simulink model "Test_Harness"  (R2018b)
settings: Solver=FixedStepAuto  StartTime=0  StopTime=300  MaxStep=0.01  RelTol=1e-4  EnableMultiTasking=on
undefined symbols (not defined in the file): actuatorCentres, aeroCoeff, datcom1, deflectionLimits, HDBK, MIL, sensorSampleTime, vehicle
libraries: arduinolib x7, aerolibasang x5, aerolibactuator x4, aerolibadyn x3, aerolibconvert2 x2, shared6dof x1, aerolibwind2 x1, aerolibatmos2 x1, pil_lib x1, aerolibanimutils x1
settings Model: DataDictionary=data.sldd  VariantConfigurationObject=Variants  SnapshotBufferSize=2  SnapshotInterval=1  PacingRate=10  ExtModeTrigDuration=2  Creator=Aliak  LastModifiedBy=Aliak
settings SolverCC: SolverResetMethod=Robust  MinimalZcImpactIntegration=on
settings OptimizationCC: DefaultParameterBehavior=Inlined  UseDivisionForNetSlopeComputation=on  UseFloatMulNetSlope=on  DefaultUnderspecifiedDataType=single  UseSpecifiedMinMax=on  InlineInvariantSignals=on  EnhancedBackFolding=on  BooleansAsBitfields=on  PassReuseOutputArgsAs=Individual arguments  StateBitsets=on  DataBitsets=on  ZeroExternalMemoryAtStartup=off  ZeroInternalMemoryAtStartup=off  NoFixptDivByZeroProtection=on  EfficientFloat2IntCast=on  LifeSpan=0.01  MaxStackSize=64  SimCompilerOptimization=on  OptimizeBlockOrder=speed  DifferentSizesBufferReuse=on
settings DebuggingCC: ConsistencyChecking=warning  ReadBeforeWriteMsg=DisableAll  WriteAfterWriteMsg=DisableAll  WriteAfterReadMsg=DisableAll  SolverPrmCheckMsg=warning  ParameterTunabilityLossMsg=error  UniqueDataStoreMsg=error  BusObjectLabelMismatch=error  StateNameClashWarn=warning  ForceCombineOutputUpdateInSim=on
settings HardwareCC: ProdBitPerInt=16  ProdBitPerPointer=16  ProdBitPerSizeT=16  ProdBitPerPtrDiffT=16  ProdLargestAtomicFloat=None  ProdWordSize=8  ProdLongLongMode=on  ProdHWDeviceType=Atmel->AVR
settings ModelReferenceCC: UpdateModelReferenceTargets=IfOutOfDate  EnableParallelModelReferenceBuilds=on  ModelReferenceMinAlgLoopOccurrences=on
settings SFSimCC: SimUserIncludeDirs="\"nativelibs/include\" \"nativelibs/src\" \"nativelibs/build\""  SFSimEcho=off  MATLABDynamicMemAlloc=off
settings RTWCC: SystemTargetFile=ert.tlc  HardwareBoard=Arduino Uno  TemplateMakefile=ert_default_tmf  GenerateReport=on  RTWUseSimCustomCode=on  CustomInclude="\"nativelibs/include\" \"nativelibs/src\" \"nativelibs/build\""  Toolchain=Arduino AVR  BuildConfiguration=Faster Runs  IncludeHyperlinkInReport=on  LaunchReport=on  PortableWordSizes=on  CreateSILPILBlock=PIL  GenerateTraceInfo=on  GenerateTraceReport=on  GenerateTraceReportSl=on  GenerateTraceReportSf=on  GenerateTraceReportEml=on  GenerateCodeMetricsReport=on
settings CodeAppCC: ForceParamTrailComments=on  IgnoreCustomStorageClasses=off  OperatorAnnotations=on  SimulinkDataObjDesc=on  SFDataObjDesc=on  CustomSymbolStrGlobalVar=rt$N$M  CustomSymbolStrType=$N$M  CustomSymbolStrFcn=$N$M$F  CustomSymbolStrMacro=$N$M  InsertBlockDesc=on
settings ERTTargetCC: TargetLangStandard=C99 (ISO)  UtilityFuncGeneration=Shared location  IncludeMdlTerminateFcn=off  CombineSignalStateStructs=on  SuppressErrorStatus=on  SupportNonFinite=off  SupportComplex=off  SupportVariableSizeSignals=on  CastingMode=Standards  ERTFilePackagingFormat=CompactWithDataFile

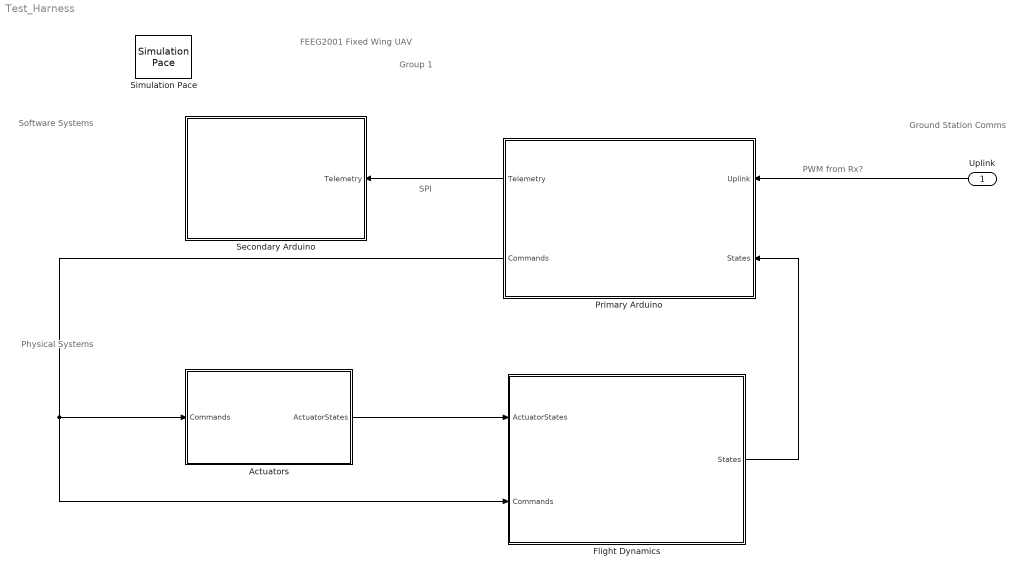
== system Test_Harness ==
  note: PWM from Rx?
  note: SPI
  note: Group 1
  note: FEEG2001 Fixed Wing UAV
  note: Physical Systems
  note: Software Systems
  note: Ground Station Comms
  Uplink : Inport  OutDataTypeStr=Bus: Uplink
  Actuators : Subsystem  Variant=on
  Flight Dynamics : Subsystem
      mask Display: image('MQ-9-Reaper-armed-UAV.jpg');
  Primary Arduino : Subsystem  DialogController=pil_create_dialog  LoadFcn=|
      | try
      |    if ~strcmp(rtw.pil.getPILVersion, '9.5 (R2018b)_13')
      |       set_param(gcb, 'DialogController', '');
      |       set_param(gcb, 'DialogControllerArgs', '');
      |    end
      | catch e
      |       set_param(gcb, 'DialogController', '');
      |       set_param(gcb, 'DialogControllerArgs', '');
      | end
      mask help: PIL:pil:XILBlockMaskDesc
      mask Display: disp('PIL');
  Secondary Arduino : Subsystem  VariantControl=Variant1
      mask Display: image('a000066_featured_1_.jpg');
  Simulation Pace : aerolibanimutils/Simulation Pace  SimulationPace=1  SleepMode=Auto  OutputPaceError=off  SampleTime=sensorSampleTime
  wires:
  Actuators/1(ActuatorStates) -> Flight Dynamics/1(ActuatorStates)
  Primary Arduino/2(Commands) -> Flight Dynamics/2(Commands), Actuators/1(Commands)
  Uplink/1 -> Primary Arduino/1(Uplink)
  Flight Dynamics/1(States) -> Primary Arduino/2(States)
  Primary Arduino/1(Telemetry) -> Secondary Arduino/1(Telemetry)

== system Test_Harness/Actuators ==
  Commands : Inport
  Model Actuators : Subsystem  VariantControl=SimType == 0
  Real Actuators : Subsystem  VariantControl=SimType == 1
  ActuatorStates : Outport

== system Test_Harness/Flight Dynamics ==
  ActuatorStates : Inport
  Commands : Inport  Port=2  OutDataTypeStr=Bus: Commands
  6DOF EOM : Subsystem  VariantControl=eom3DOF
  Bus Selector : BusSelector  OutputSignals=Throttle
  Coeff Model : Subsystem  Commented=on  VariantControl=AeroModel==2
  DATCOM Model : Subsystem  VariantControl=AeroModel==1
  Environment : Subsystem
  Propulsion : Subsystem
      settings: RTWSystemCode=Inline
  Sum1 : Sum  Inputs=|++  SaturateOnIntegerOverflow=on  InputSameDT=on  OutDataTypeStr=Inherit: Same as first input
  Sum2 : Sum  Inputs=|++  SaturateOnIntegerOverflow=on  InputSameDT=on  OutDataTypeStr=Inherit: Same as first input
  Visualization : Subsystem
  States : Outport
  wires:
  Commands/1 -> Bus Selector/1
  Sum2/1 -> 6DOF EOM/2(Forces)
  Propulsion/1(F) -> Sum2/2
  Propulsion/2(M) -> Sum1/2
  Sum1/1 -> 6DOF EOM/3(Moments)
  Bus Selector/1 -> Propulsion/1(cmd)  "<Throttle>"
  ActuatorStates/1 -> DATCOM Model/3(ActuatorStates)
  DATCOM Model/1(F) -> Sum2/1
  DATCOM Model/2(M) -> Sum1/1
  Environment/1(Env) -> 6DOF EOM/1(Env), DATCOM Model/1(Env)
  6DOF EOM/1(DCMbe) -> Environment/2(DCMbe)
  6DOF EOM/2(States) -> Environment/1(States), Visualization/1(States), DATCOM Model/2(States), States/1

== system Test_Harness/Primary Arduino ==
  Uplink : Inport  OutDataTypeStr=Bus: Uplink
  States : Inport  Port=2
  Primary Arduino_sfcn : pil_lib/PIL Block  SimulationMode=PIL  IsTopModelPIL=off  CodeDir=D:\MATLABProjects\FEEG2001-FWUAV\libs\Primary_ert_rtw  AnchorDir=D:\MATLABProjects\FEEG2001-FWUAV\libs  ConfigName=Arduino Board  XrelIsTopModelCode=on  XrelIsReusable=off  XrelDWorkNames={}  XrelDWorkTypes={}  XrelModelArgVals={}  XrelOrderedParamNames={}
  __InputSSForSFun__ : Subsystem
  __OutputSSForSFun__ : Subsystem
  Telemetry : Outport  OutDataTypeStr=Bus: Sensors  SampleTime=[1 0]
  Commands : Outport  Port=2  OutDataTypeStr=Bus: Commands  SampleTime=[-1 0]
  wires:
  Uplink/1 -> __InputSSForSFun__/1(Uplink)
  States/1 -> __InputSSForSFun__/2(States)
  __InputSSForSFun__/1(__UniqueOutportName__1__) -> Primary Arduino_sfcn/1
  __InputSSForSFun__/2(__UniqueOutportName__2__) -> Primary Arduino_sfcn/2
  __InputSSForSFun__/3(__UniqueOutportName__3__) -> Primary Arduino_sfcn/3
  __InputSSForSFun__/4(__UniqueOutportName__4__) -> Primary Arduino_sfcn/4
  __InputSSForSFun__/5(__UniqueOutportName__5__) -> Primary Arduino_sfcn/5
  __InputSSForSFun__/6(__UniqueOutportName__6__) -> Primary Arduino_sfcn/6
  __InputSSForSFun__/7(__UniqueOutportName__7__) -> Primary Arduino_sfcn/7
  Primary Arduino_sfcn/1 -> __OutputSSForSFun__/1(__UniqueInportName__1__)
  Primary Arduino_sfcn/2 -> __OutputSSForSFun__/2(__UniqueInportName__2__)
  __OutputSSForSFun__/1(Telemetry) -> Telemetry/1
  __OutputSSForSFun__/2(Commands) -> Commands/1

== system Test_Harness/Secondary Arduino ==
  Telemetry : Inport
  Telemetry Logging : Subsystem  VariantControlMode=Label  Variant=on  VariantControl=Variant1  LabelModeActiveChoice=SecArd==0
  wires:
  Telemetry/1 -> Telemetry Logging/1("Telemetry ")

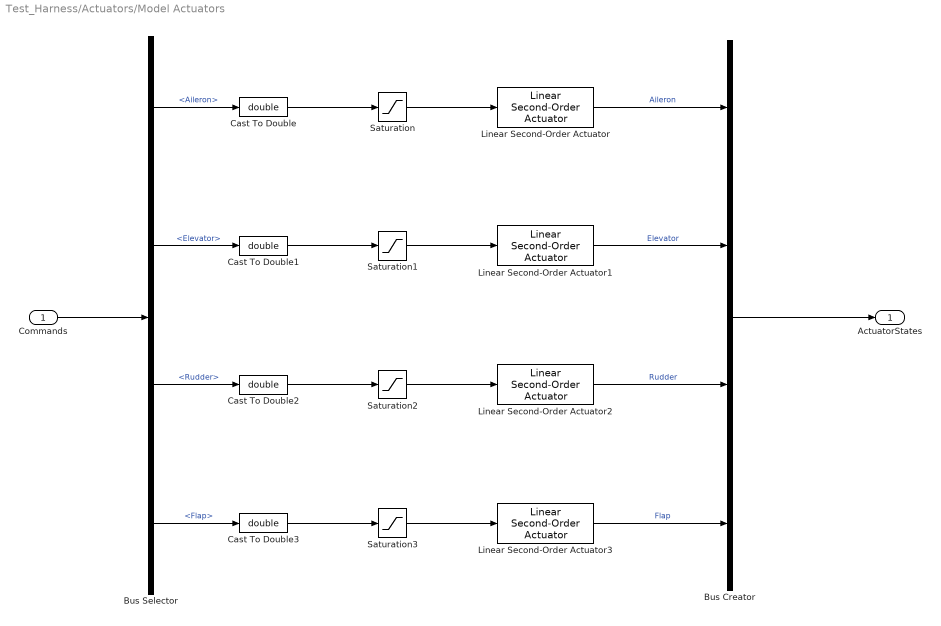
== system Test_Harness/Actuators/Model Actuators ==
  Commands : Inport
  Bus Creator : BusCreator  Inputs=4  OutDataTypeStr=Bus: ActuatorStates
  Bus Selector : BusSelector  OutputSignals=Aileron,Elevator,Rudder,Flap
  Cast To Double{,1..3} (4 alike) : DataTypeConversion  OutDataTypeStr=double
  Linear Second-Order Actuator{,1..3} (4 alike) : aerolibactuator/Linear Second-Order Actuator  wn_fin=1  z_fin=0.3  fin_act_0=0  fin_act_vel=0
      settings: SourceProductName=Aerospace Blockset  SourceProductBaseCode=AE
  Saturation : Saturate  UpperLimit=deflectionLimits.aileron.max  LowerLimit=deflectionLimits.aileron.min
  Saturation1 : Saturate  UpperLimit=deflectionLimits.elevator.max  LowerLimit=deflectionLimits.elevator.min
  Saturation2 : Saturate  UpperLimit=deflectionLimits.rudder.max  LowerLimit=deflectionLimits.rudder.min
  Saturation3 : Saturate  UpperLimit=deflectionLimits.flap.max  LowerLimit=deflectionLimits.flap.min
  ActuatorStates : Outport
  wires:
  Bus Selector/3 -> Cast To Double2/1  "<Rudder>"
  Bus Selector/4 -> Cast To Double3/1  "<Flap>"
  Bus Selector/1 -> Cast To Double/1  "<Aileron>"
  Bus Selector/2 -> Cast To Double1/1  "<Elevator>"
  Saturation/1 -> Linear Second-Order Actuator/1
  Saturation1/1 -> Linear Second-Order Actuator1/1
  Saturation2/1 -> Linear Second-Order Actuator2/1
  Saturation3/1 -> Linear Second-Order Actuator3/1
  Linear Second-Order Actuator1/1 -> Bus Creator/2  "Elevator"
  Linear Second-Order Actuator/1 -> Bus Creator/1  "Aileron"
  Linear Second-Order Actuator2/1 -> Bus Creator/3  "Rudder"
  Linear Second-Order Actuator3/1 -> Bus Creator/4  "Flap"
  Bus Creator/1 -> ActuatorStates/1
  Commands/1 -> Bus Selector/1
  Cast To Double/1 -> Saturation/1
  Cast To Double1/1 -> Saturation1/1
  Cast To Double2/1 -> Saturation2/1
  Cast To Double3/1 -> Saturation3/1

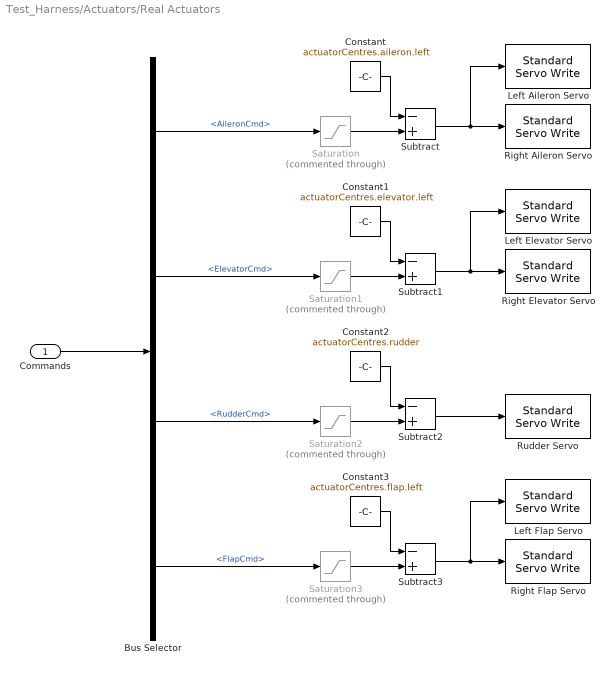
== system Test_Harness/Actuators/Real Actuators ==
  Commands : Inport
  Bus Selector : BusSelector  OutputSignals=AileronCmd,ElevatorCmd,RudderCmd,FlapCmd
  Constant : Constant  Value=actuatorCentres.aileron.left
  Constant1 : Constant  Value=actuatorCentres.elevator.left
  Constant2 : Constant  Value=actuatorCentres.rudder
  Constant3 : Constant  Value=actuatorCentres.flap.left
  Left Aileron Servo : arduinolib/Standard Servo Write  pinNumber=servoPins.aileron.left  ServoIndex=0  blockPlatform=ARDUINO
      settings: SourceProductName=Simulink Support Package for Arduino Hardware
  Left Elevator Servo : arduinolib/Standard Servo Write  pinNumber=servoPins.elevator.left  ServoIndex=0  blockPlatform=ARDUINO
      settings: SourceProductName=Simulink Support Package for Arduino Hardware
  Left Flap Servo : arduinolib/Standard Servo Write  pinNumber=servoPins.flap.left  ServoIndex=0  blockPlatform=ARDUINO
      settings: SourceProductName=Simulink Support Package for Arduino Hardware
  Right Aileron Servo : arduinolib/Standard Servo Write  pinNumber=servoPins.aileron.right  ServoIndex=0  blockPlatform=ARDUINO
      settings: SourceProductName=Simulink Support Package for Arduino Hardware
  Right Elevator Servo : arduinolib/Standard Servo Write  pinNumber=servoPins.elevator.right  ServoIndex=0  blockPlatform=ARDUINO
      settings: SourceProductName=Simulink Support Package for Arduino Hardware
  Right Flap Servo : arduinolib/Standard Servo Write  pinNumber=servoPins.flap.right  ServoIndex=0  blockPlatform=ARDUINO
      settings: SourceProductName=Simulink Support Package for Arduino Hardware
  Rudder Servo : arduinolib/Standard Servo Write  pinNumber=servoPins.rudder  ServoIndex=0  blockPlatform=ARDUINO
      settings: SourceProductName=Simulink Support Package for Arduino Hardware
  Saturation : Saturate  Commented=through  UpperLimit=deflectionLimits.aileron.max  LowerLimit=deflectionLimits.aileron.min
  Saturation1 : Saturate  Commented=through  UpperLimit=deflectionLimits.elevator.max  LowerLimit=deflectionLimits.elevator.min
  Saturation2 : Saturate  Commented=through  UpperLimit=deflectionLimits.rudder.max  LowerLimit=deflectionLimits.rudder.min
  Saturation3 : Saturate  Commented=through  UpperLimit=deflectionLimits.flap.max  LowerLimit=deflectionLimits.flap.min
  Subtract{,1..3} (4 alike) : Sum  Inputs=-+
  wires:
  Saturation/1 -> Subtract/2
  Bus Selector/3 -> Saturation2/1  "<RudderCmd>"
  Commands/1 -> Bus Selector/1
  Bus Selector/4 -> Saturation3/1  "<FlapCmd>"
  Subtract3/1 -> Right Flap Servo/1, Left Flap Servo/1
  Bus Selector/1 -> Saturation/1  "<AileronCmd>"
  Constant2/1 -> Subtract2/1
  Subtract2/1 -> Rudder Servo/1
  Saturation3/1 -> Subtract3/2
  Saturation2/1 -> Subtract2/2
  Saturation1/1 -> Subtract1/2
  Bus Selector/2 -> Saturation1/1  "<ElevatorCmd>"
  Subtract/1 -> Right Aileron Servo/1, Left Aileron Servo/1
  Subtract1/1 -> Right Elevator Servo/1, Left Elevator Servo/1
  Constant/1 -> Subtract/1
  Constant1/1 -> Subtract1/1
  Constant3/1 -> Subtract3/1

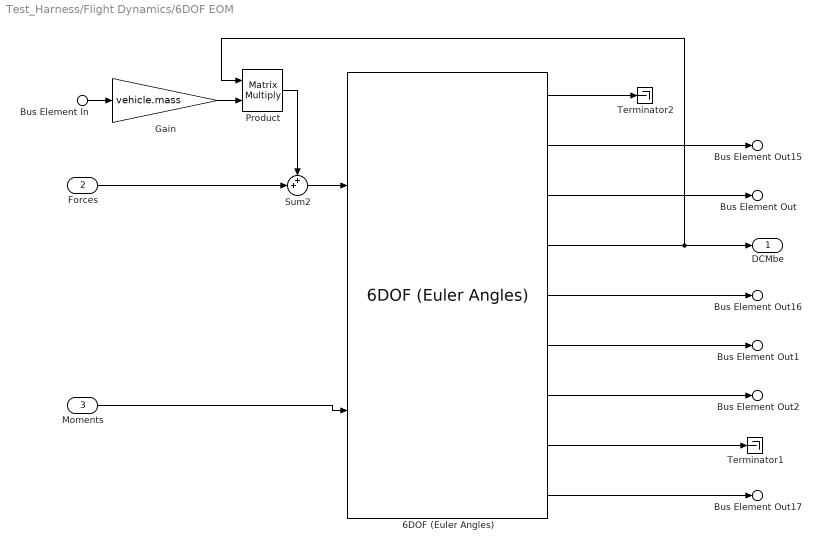
== system Test_Harness/Flight Dynamics/6DOF EOM ==
  Bus Element In : Inport  PortName=Env  Element=g
  Forces : Inport  Port=2
  Moments : Inport  Port=3
  6DOF (Euler Angles) : shared6dof/6DOF (Euler Angles)  units=Metric (MKS)  mtype=Fixed  rep=Euler Angles  xme_0=initConditions.x0  Vm_0=initConditions.v0  eul_0=initConditions.euler0  pm_0=initConditions.w0  mass_0=vehicle.mass  mass_e=0.5  mass_f=2.0  inertia=vehicle.inertia  inertia_e=eye(3)  inertia_f=2*eye(3)  k_quat=1.0  vre_flag=on  abi_flag=on  aMode=0  xme_statename=''  Vm_statename=''  eul_statename=''  quat_statename=''  pm_statename=''  mass_statename=''
      settings: SourceProductBaseCode=AE
  Gain : Gain  Gain=vehicle.mass
  Product : Product  Multiplication=Matrix(*)
  Sum2 : Sum  Inputs=++|  SaturateOnIntegerOverflow=on  InputSameDT=on  OutDataTypeStr=Inherit: Same as first input
  Terminator1 : Terminator
  Terminator2 : Terminator
  DCMbe : Outport
  Bus Element Out : Outport  Port=2  PortName=States  Element=phi_theta_psi
  Bus Element Out1 : Outport  Port=2  PortName=States  Element=pqr
  Bus Element Out2 : Outport  Port=2  PortName=States  Element=omega_dot
  Bus Element Out15 : Outport  Port=2  PortName=States  Element=X_e
  Bus Element Out16 : Outport  Port=2  PortName=States  Element=V_b
  Bus Element Out17 : Outport  Port=2  PortName=States  Element=A_be
  wires:
  6DOF (Euler Angles)/4 -> DCMbe/1, Product/1
  6DOF (Euler Angles)/1 -> Terminator2/1
  Bus Element In/1 -> Gain/1
  6DOF (Euler Angles)/9 -> Bus Element Out17/1
  6DOF (Euler Angles)/7 -> Bus Element Out2/1
  6DOF (Euler Angles)/6 -> Bus Element Out1/1
  6DOF (Euler Angles)/5 -> Bus Element Out16/1
  6DOF (Euler Angles)/3 -> Bus Element Out/1
  6DOF (Euler Angles)/2 -> Bus Element Out15/1
  Gain/1 -> Product/2
  Sum2/1 -> 6DOF (Euler Angles)/1
  Product/1 -> Sum2/1
  6DOF (Euler Angles)/8 -> Terminator1/1
  Moments/1 -> 6DOF (Euler Angles)/2
  Forces/1 -> Sum2/2

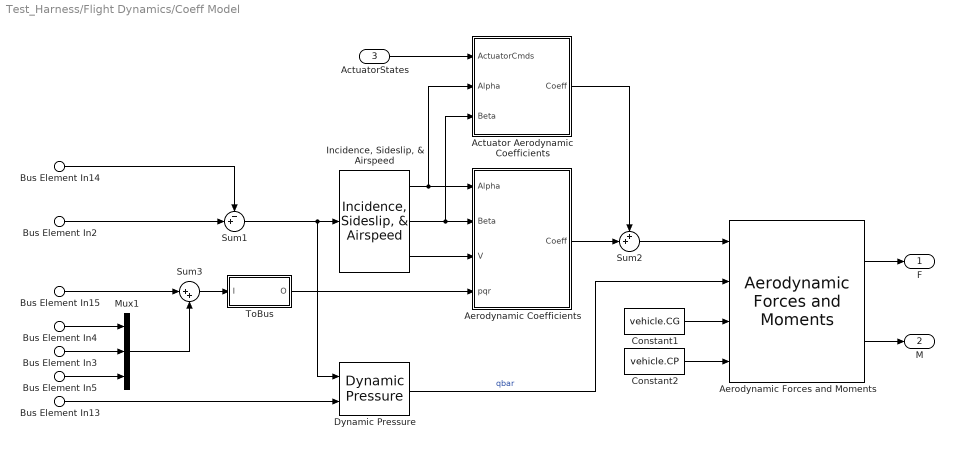
== system Test_Harness/Flight Dynamics/Coeff Model ==
  Bus Element In13 : Inport  PortName=Env  Element=AirDensity
  Bus Element In14 : Inport  PortName=Env  Element=WindVelocity
  Bus Element In15 : Inport  PortName=Env  Element=WindAngularRates
  Bus Element In3 : Inport  Port=2  PortName=States  Element=q
  Bus Element In4 : Inport  Port=2  PortName=States  Element=p
  Bus Element In5 : Inport  Port=2  PortName=States  Element=r
  Bus Element In2 : Inport  Port=2  PortName=States  Element=V_b
  ActuatorStates : Inport  Port=3  OutDataTypeStr=Bus: ActuatorStates
  Actuator Aerodynamic Coefficients : Subsystem
  Aerodynamic Coefficients : Subsystem
  Aerodynamic Forces and Moments : aerolibadyn/Aerodynamic Forces and Moments   inputAxes=Body  outputForceAxes=Body  outputMomentAxes=Body  S=vehicle.wingarea  b=vehicle.wingspan  cbar=vehicle.aclength
      settings: SourceProductName=Aerospace Blockset
  Constant1 : Constant  Value=vehicle.CG
  Constant2 : Constant  Value=vehicle.CP
  Dynamic Pressure : aerolibasang/Dynamic Pressure
  "Incidence, Sideslip, & Airspeed" : aerolibasang/Incidence, Sideslip, & Airspeed
      settings: SourceProductName=Aerospace Blockset
  Mux1 : Mux  Inputs=3
  Sum1 : Sum  Inputs=-+|  SaturateOnIntegerOverflow=on  InputSameDT=on  OutDataTypeStr=Inherit: Same as first input
  Sum2 : Sum  Inputs=++|
  Sum3 : Sum  Inputs=|++  SaturateOnIntegerOverflow=on  InputSameDT=on  OutDataTypeStr=Inherit: Same as first input
  ToBus : Subsystem
  F : Outport  Unit=N
  M : Outport  Port=2  Unit=N*m
  wires:
  ActuatorStates/1 -> Actuator Aerodynamic Coefficients/1(ActuatorCmds)
  Bus Element In14/1 -> Sum1/1
  Bus Element In2/1 -> Sum1/2
  Mux1/1 -> Sum3/2
  Bus Element In15/1 -> Sum3/1
  Bus Element In5/1 -> Mux1/3
  Bus Element In3/1 -> Mux1/2
  Bus Element In4/1 -> Mux1/1
  Actuator Aerodynamic Coefficients/1(Coeff) -> Sum2/1
  Aerodynamic Coefficients/1(Coeff) -> Sum2/2
  ToBus/1(O) -> Aerodynamic Coefficients/4(pqr)
  Sum1/1 -> Dynamic Pressure/1, "Incidence, Sideslip, & Airspeed"/1
  Dynamic Pressure/1 -> Aerodynamic Forces and Moments/2  "qbar"
  Sum3/1 -> ToBus/1(I)
  Bus Element In13/1 -> Dynamic Pressure/2
  "Incidence, Sideslip, & Airspeed"/3 -> Aerodynamic Coefficients/3(V)
  "Incidence, Sideslip, & Airspeed"/2 -> Aerodynamic Coefficients/2(Beta), Actuator Aerodynamic Coefficients/3(Beta)
  Aerodynamic Forces and Moments/2 -> M/1
  Aerodynamic Forces and Moments/1 -> F/1
  Constant2/1 -> Aerodynamic Forces and Moments/4
  Constant1/1 -> Aerodynamic Forces and Moments/3
  Sum2/1 -> Aerodynamic Forces and Moments/1
  "Incidence, Sideslip, & Airspeed"/1 -> Actuator Aerodynamic Coefficients/2(Alpha), Aerodynamic Coefficients/1(Alpha)

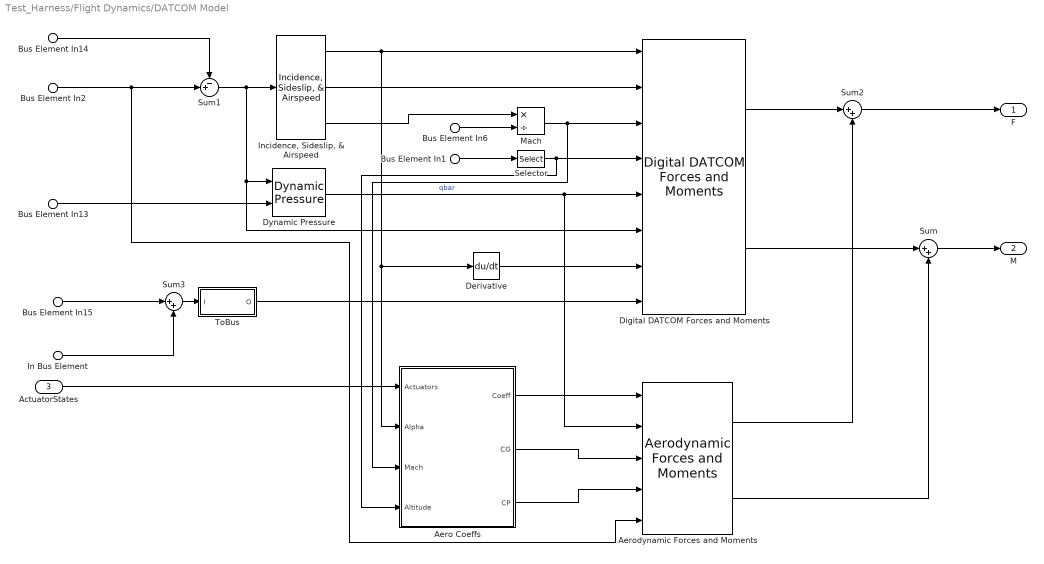
== system Test_Harness/Flight Dynamics/DATCOM Model ==
  Bus Element In13 : Inport  PortName=Env  Element=AirDensity
  Bus Element In14 : Inport  PortName=Env  Element=WindVelocity
  Bus Element In15 : Inport  PortName=Env  Element=WindAngularRates
  Bus Element In6 : Inport  PortName=Env  Element=a
  Bus Element In2 : Inport  Port=2  PortName=States  Element=V_b
  Bus Element In1 : Inport  Port=2  PortName=States  Element=X_e
  In Bus Element : Inport  Port=2  PortName=States  Element=pqr
  ActuatorStates : Inport  Port=3  OutDataTypeStr=Bus: ActuatorStates
  Aero Coeffs : Subsystem
  "Aerodynamic Forces and Moments " : aerolibadyn/Aerodynamic Forces and Moments   inputAxes=Stability  outputForceAxes=Body  outputMomentAxes=Body  S=vehicle.wingarea  b=vehicle.wingspan  cbar=vehicle.cbar
      settings: SourceProductName=Aerospace Blockset
  Derivative : Derivative
  Digital DATCOM Forces and Moments : aerolibadyn/Digital DATCOM Forces and Moments  units=Metric (MKS)  dcase=datcom1{3}  fmode=Body  buildno=0  imethod=Linear  emethod=Linear  rmethod=Linear Extrapolation  action=Warning
      settings: SourceProductName=Aerospace Blockset  SourceProductBaseCode=AE
  Dynamic Pressure : aerolibasang/Dynamic Pressure
  "Incidence, Sideslip, & Airspeed" : aerolibasang/Incidence, Sideslip, & Airspeed
      settings: SourceProductName=Aerospace Blockset
  Mach : Product  Inputs=*/
  Selector : Selector  IndexMode=Zero-based  InputPortWidth=3  IndexOptions=Index vector (dialog)  Indices=[2]  OutputSizes=1
  Sum : Sum  Inputs=|++
  Sum1 : Sum  Inputs=-+|  SaturateOnIntegerOverflow=on  InputSameDT=on  OutDataTypeStr=Inherit: Same as first input
  Sum2 : Sum  Inputs=|++
  Sum3 : Sum  Inputs=|++  SaturateOnIntegerOverflow=on  InputSameDT=on  OutDataTypeStr=Inherit: Same as first input
  ToBus : Subsystem
  F : Outport  Unit=N
  M : Outport  Port=2  Unit=N*m
  wires:
  Bus Element In14/1 -> Sum1/1
  Bus Element In2/1 -> "Aerodynamic Forces and Moments "/5, Sum1/2
  In Bus Element/1 -> Sum3/2
  Bus Element In15/1 -> Sum3/1
  Sum1/1 -> "Incidence, Sideslip, & Airspeed"/1, Digital DATCOM Forces and Moments/6, Dynamic Pressure/1
  Sum3/1 -> ToBus/1(I)
  Bus Element In13/1 -> Dynamic Pressure/2
  "Incidence, Sideslip, & Airspeed"/3 -> Mach/1
  Digital DATCOM Forces and Moments/2 -> Sum/1
  Digital DATCOM Forces and Moments/1 -> Sum2/1
  Dynamic Pressure/1 -> "Aerodynamic Forces and Moments "/2, Digital DATCOM Forces and Moments/5  "qbar"
  Bus Element In1/1 -> Selector/1
  Selector/1 -> Aero Coeffs/4(Altitude), Digital DATCOM Forces and Moments/4
  Bus Element In6/1 -> Mach/2
  ActuatorStates/1 -> Aero Coeffs/1(Actuators)
  "Incidence, Sideslip, & Airspeed"/2 -> Digital DATCOM Forces and Moments/2
  "Incidence, Sideslip, & Airspeed"/1 -> Digital DATCOM Forces and Moments/1, Derivative/1, Aero Coeffs/2(Alpha)
  Aero Coeffs/1(Coeff) -> "Aerodynamic Forces and Moments "/1
  Aero Coeffs/2(CG) -> "Aerodynamic Forces and Moments "/3
  Aero Coeffs/3(CP) -> "Aerodynamic Forces and Moments "/4
  Sum/1 -> M/1
  "Aerodynamic Forces and Moments "/2 -> Sum/2
  Sum2/1 -> F/1
  "Aerodynamic Forces and Moments "/1 -> Sum2/2
  ToBus/1(O) -> Digital DATCOM Forces and Moments/8
  Derivative/1 -> Digital DATCOM Forces and Moments/7
  Mach/1 -> Digital DATCOM Forces and Moments/3, Aero Coeffs/3(Mach)

== system Test_Harness/Flight Dynamics/Environment ==
  States : Inport
  DCMbe : Inport  Port=2
  Bus Creator : BusCreator  Inputs=5
  Bus Selector : BusSelector  OutputSignals=X_e,V_b
  Dryden Wind Turbulence Model (Discrete (-q +r)) : aerolibwind2/Dryden Wind Turbulence Model  (Continuous (+q -r))  units=Metric (MKS)  spec=MIL-HDBK-1797  model=Discrete Dryden (-q +r)  W20=1  Wdeg=250  TurbProb=10^-1  L_high=533.4  Wingspan=1.8  ts=sensorSampleTime  Seed=[23341 23342 23343 23344]  T_on=off
      settings: SourceProductName=Aerospace Blockset
  Lapse Rate Model : aerolibatmos2/ISA Atmosphere Model  custom=off  g=9.80665  gamma=1.4  R=287.0531  L=0.0065  h_trop=11000  h_strat=20000  rho0=1.225  P0=101325  T0=288.15  h0=0
      settings: SourceProductName=Aerospace Blockset
  Selector : Selector  IndexMode=Zero-based  InputPortWidth=3  IndexOptions=Index vector (dialog)  Indices=[0]  OutputSizes=1
  Selector1 : Selector  IndexMode=Zero-based  InputPortWidth=3  IndexOptions=Index vector (dialog)  Indices=[0]  OutputSizes=1
  Terminator : Terminator
  Terminator1 : Terminator
  g : Constant  Value=[0 0 9.80665]
  Env : Outport
  wires:
  States/1 -> Bus Selector/1
  Bus Creator/1 -> Env/1
  Selector/1 -> Dryden Wind Turbulence Model (Discrete (-q +r))/1, Lapse Rate Model/1
  Bus Selector/1 -> Selector/1  "<X_e>"
  Lapse Rate Model/4 -> Bus Creator/2  "AirDensity"
  Lapse Rate Model/2 -> Bus Creator/1  "a"
  g/1 -> Bus Creator/3  "g"
  DCMbe/1 -> Dryden Wind Turbulence Model (Discrete (-q +r))/3
  Bus Selector/2 -> Selector1/1  "<V_b>"
  Selector1/1 -> Dryden Wind Turbulence Model (Discrete (-q +r))/2
  Dryden Wind Turbulence Model (Discrete (-q +r))/1 -> Bus Creator/4  "WindVelocity"
  Dryden Wind Turbulence Model (Discrete (-q +r))/2 -> Bus Creator/5  "WindAngularRates"
  Lapse Rate Model/1 -> Terminator/1
  Lapse Rate Model/3 -> Terminator1/1

== system Test_Harness/Flight Dynamics/Propulsion ==
  cmd : Inport  OutDataTypeStr=single
  Cast To Double : DataTypeConversion  OutDataTypeStr=double
  Mux : Mux  Inputs=[1 2]
  Product : Product
  ThrustX : Lookup_n-D  NumberOfTableDimensions=1  LookupTableObject=''  BreakpointsForDimension1=(1/6)*(3+([-3:3]))  IndexSearchMethod=Linear search  BeginIndexSearchUsingPreviousIndexResult=on  Table=vehicle.thrust*(1+tanh([-3:3]))  ExtrapMethod=Clip  InternalRulePriority=Speed
  ThrustYZ : Constant  Value=[0 0]'  SampleTime=-1
  Thrust_M1 : Constant  Value=[-0.1 0 0.01]  SampleTime=-1
  Vector Concatenate : Concatenate
  F : Outport  Unit=N
  M : Outport  Port=2  Unit=N*m
  wires:
  Thrust_M1/1 -> Product/2
  ThrustX/1 -> Mux/1, Vector Concatenate/2
  ThrustYZ/1 -> Vector Concatenate/1, Mux/2
  Mux/1 -> F/1
  cmd/1 -> Cast To Double/1
  Product/1 -> M/1
  Vector Concatenate/1 -> Product/1
  Cast To Double/1 -> ThrustX/1

== system Test_Harness/Flight Dynamics/Visualization ==
  Bus Element In3 : Inport  PortName=States  Element=pqr
  Bus Element In9 : Inport  PortName=States  Element=X_e
  In Bus Element : Inport  PortName=States  Element=V_b
  In Bus Element1 : Inport  PortName=States  Element=phi_theta_psi
  "Incidence, Sideslip, & Airspeed" : aerolibasang/Incidence, Sideslip, & Airspeed
      settings: SourceProductName=Aerospace Blockset
  Mux5 : Mux  Inputs=2
  State Plots : Scope  NumInputPorts=4
  Terminator : Terminator
  wires:
  Bus Element In9/1 -> State Plots/4
  In Bus Element1/1 -> State Plots/2
  Mux5/1 -> State Plots/1
  "Incidence, Sideslip, & Airspeed"/2 -> Mux5/2  "beta"
  "Incidence, Sideslip, & Airspeed"/1 -> Mux5/1  "alpha"
  In Bus Element/1 -> "Incidence, Sideslip, & Airspeed"/1
  Bus Element In3/1 -> State Plots/3
  "Incidence, Sideslip, & Airspeed"/3 -> Terminator/1

== system Test_Harness/Primary Arduino/__InputSSForSFun__ ==
  Uplink : Inport  OutDataTypeStr=Bus: Uplink
  States : Inport  Port=2
  temporaryBusSelectName_1 : BusSelector  OutputSignals=phi_theta_psi,pqr,omega_dot,X_e,V_b,A_be
  __UniqueOutportName__1__ : Outport
  __UniqueOutportName__2__ : Outport  Port=2
  __UniqueOutportName__3__ : Outport  Port=3
  __UniqueOutportName__4__ : Outport  Port=4
  __UniqueOutportName__5__ : Outport  Port=5
  __UniqueOutportName__6__ : Outport  Port=6
  __UniqueOutportName__7__ : Outport  Port=7
  wires:
  States/1 -> temporaryBusSelectName_1/1
  Uplink/1 -> __UniqueOutportName__1__/1
  temporaryBusSelectName_1/1 -> __UniqueOutportName__2__/1  "<phi_theta_psi>"
  temporaryBusSelectName_1/2 -> __UniqueOutportName__3__/1  "<pqr>"
  temporaryBusSelectName_1/3 -> __UniqueOutportName__4__/1  "<omega_dot>"
  temporaryBusSelectName_1/4 -> __UniqueOutportName__5__/1  "<X_e>"
  temporaryBusSelectName_1/5 -> __UniqueOutportName__6__/1  "<V_b>"
  temporaryBusSelectName_1/6 -> __UniqueOutportName__7__/1  "<A_be>"

== system Test_Harness/Primary Arduino/__OutputSSForSFun__ ==
  __UniqueInportName__1__ : Inport
  __UniqueInportName__2__ : Inport  Port=2
  Telemetry : Outport  OutDataTypeStr=Bus: Sensors  SampleTime=[1 0]
  Commands : Outport  Port=2  OutDataTypeStr=Bus: Commands  SampleTime=[-1 0]
  wires:
  __UniqueInportName__1__/1 -> Telemetry/1
  __UniqueInportName__2__/1 -> Commands/1

== system Test_Harness/Secondary Arduino/Telemetry Logging ==
  "Telemetry " : Inport
  SD Logging : Subsystem  VariantControl=SecArd==1
  Simulink Logging : Subsystem  VariantControl=SecArd==0

== system Test_Harness/Flight Dynamics/Coeff Model/Actuator Aerodynamic Coefficients ==
  Bus Element In13 : Inport  PortName=ActuatorCmds  Element=Elevator
  Bus Element In1 : Inport  PortName=ActuatorCmds  Element=Aileron
  Bus Element In2 : Inport  PortName=ActuatorCmds  Element=Rudder
  Alpha : Inport  Port=2
  Beta : Inport  Port=3
  Aileron : Subsystem
  Constant : Constant  Value=0
  Elevator : Subsystem
  Flap : Subsystem
  Rudder : Subsystem
  Sum : Sum  Inputs=4  SaturateOnIntegerOverflow=on  InputSameDT=on  OutDataTypeStr=Inherit: Same as first input
  Coeff : Outport  InitialOutput=0
  wires:
  Constant/1 -> Flap/1(Actuator)
  Bus Element In2/1 -> Rudder/1(Actuator)
  Bus Element In1/1 -> Aileron/1(Actuator)
  Bus Element In13/1 -> Elevator/1(Actuator)
  Beta/1 -> Elevator/2(Beta)
  Flap/1(delCoeff) -> Sum/4
  Alpha/1 -> Flap/2(Alpha), Rudder/2(Alpha), Aileron/2(Alpha)
  Rudder/1(delCoeff) -> Sum/3
  Aileron/1(delCoeff) -> Sum/2
  Elevator/1(delCoeff) -> Sum/1
  Sum/1 -> Coeff/1

== system Test_Harness/Flight Dynamics/Coeff Model/Aerodynamic Coefficients ==
  Alpha : Inport
  Beta : Inport  Port=2
  V : Inport  Port=3
  pqr : Inport  Port=4  Unit=m/s
  Body Rate Damping : Subsystem
  Datum Coefficients : Subsystem
  Sum : Sum  Inputs=|++
  Coeff : Outport
  wires:
  pqr/1 -> Body Rate Damping/2(pqr)
  Sum/1 -> Coeff/1
  V/1 -> Body Rate Damping/1(V)
  Body Rate Damping/1(Coeff) -> Sum/2
  Datum Coefficients/1(Coeff) -> Sum/1
  Beta/1 -> Datum Coefficients/2(Beta)
  Alpha/1 -> Datum Coefficients/1(Alpha)

== system Test_Harness/Flight Dynamics/Coeff Model/ToBus ==
  I : Inport
  Bus Creator3 : BusCreator  Inputs=3
  Demux : Demux  Outputs=3
  O : Outport
  wires:
  I/1 -> Demux/1
  Demux/2 -> Bus Creator3/2  "q_wind"
  Bus Creator3/1 -> O/1
  Demux/3 -> Bus Creator3/3  "r_wind"
  Demux/1 -> Bus Creator3/1  "p_wind"

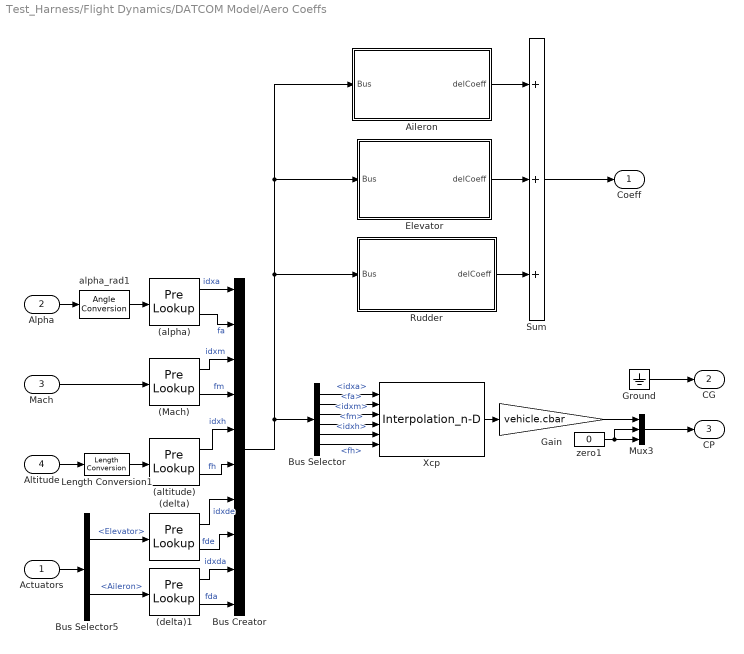
== system Test_Harness/Flight Dynamics/DATCOM Model/Aero Coeffs ==
  Actuators : Inport
  Alpha : Inport  Port=2
  Mach : Inport  Port=3
  Altitude : Inport  Port=4
  (Mach) : PreLookup  BreakpointsData=datcom1{3}.mach  BeginIndexSearchUsingPreviousIndexResult=on  ExtrapMethod=Linear  IndexDataTypeStr=int32  FractionDataTypeStr=double
  (alpha) : PreLookup  BreakpointsData=datcom1{3}.alpha  BeginIndexSearchUsingPreviousIndexResult=on  ExtrapMethod=Linear  IndexDataTypeStr=int32  FractionDataTypeStr=double
  (altitude) : PreLookup  BreakpointsData=datcom1{3}.alt  BeginIndexSearchUsingPreviousIndexResult=on  ExtrapMethod=Linear  IndexDataTypeStr=int32  FractionDataTypeStr=double
  (delta) : PreLookup  BreakpointsData=datcom1{3}.delta  BeginIndexSearchUsingPreviousIndexResult=on  ExtrapMethod=Linear  IndexDataTypeStr=int32  FractionDataTypeStr=double
  (delta)1 : PreLookup  BreakpointsData=datcom1{2}.deltal  BeginIndexSearchUsingPreviousIndexResult=on  ExtrapMethod=Linear  IndexDataTypeStr=int32  FractionDataTypeStr=double
  Aileron : Subsystem
  Bus Creator : BusCreator  Inputs=10
  Bus Selector : BusSelector  OutputSignals=idxa,fa,idxm,fm,idxh,fh
  Bus Selector5 : BusSelector  OutputSignals=Elevator,Aileron
  Elevator : Subsystem
  Gain : Gain  Gain=vehicle.cbar
  Ground : Ground
  Length Conversion1 : aerolibconvert2/Length Conversion  IU=m  OU=ft
  Mux3 : Mux  Inputs=3
  Rudder : Subsystem
  Sum : Sum  Inputs=3  SaturateOnIntegerOverflow=on  InputSameDT=on  OutDataTypeStr=Inherit: Same as first input
  Xcp : Interpolation_n-D  NumberOfTableDimensions=3  Table="permute(datcom1{1}.xcp,[1  2  3])"  OutDataTypeStr=double
      settings: InputPortMap=u0,u1,u2,u3,u4,u5
  alpha_rad1 : aerolibconvert2/Angle Conversion  IU=rad  OU=deg
  zero1 : Constant  Value=0
  Coeff : Outport
  CG : Outport  Port=2  PortDimensions=3
  CP : Outport  Port=3  PortDimensions=3
  wires:
  Aileron/1(delCoeff) -> Sum/1
  Sum/1 -> Coeff/1
  (alpha)/1 -> Bus Creator/1  "idxa"
  Gain/1 -> Mux3/1
  (delta)/2 -> Bus Creator/8  "fde"
  (alpha)/2 -> Bus Creator/2  "fa"
  Bus Selector/5 -> Xcp/5  "<idxh>"
  alpha_rad1/1 -> (alpha)/1
  Elevator/1(delCoeff) -> Sum/2
  Alpha/1 -> alpha_rad1/1
  Bus Selector/4 -> Xcp/4  "<fm>"
  Bus Selector/3 -> Xcp/3  "<idxm>"
  Mach/1 -> (Mach)/1
  (delta)/1 -> Bus Creator/7  "idxde"
  zero1/1 -> Mux3/2, Mux3/3
  Length Conversion1/1 -> (altitude)/1
  Bus Selector/1 -> Xcp/1  "<idxa>"
  Bus Creator/1 -> Bus Selector/1, Aileron/1(Bus), Elevator/1(Bus), Rudder/1(Bus)
  Bus Selector/2 -> Xcp/2  "<fa>"
  Actuators/1 -> Bus Selector5/1
  (Mach)/1 -> Bus Creator/3  "idxm"
  (Mach)/2 -> Bus Creator/4  "fm"
  Rudder/1(delCoeff) -> Sum/3
  Altitude/1 -> Length Conversion1/1
  Ground/1 -> CG/1
  Mux3/1 -> CP/1
  (altitude)/2 -> Bus Creator/6  "fh"
  (altitude)/1 -> Bus Creator/5  "idxh"
  Xcp/1 -> Gain/1
  Bus Selector5/1 -> (delta)/1  "<Elevator>"
  Bus Selector/6 -> Xcp/6  "<fh>"
  Bus Selector5/2 -> (delta)1/1  "<Aileron>"
  (delta)1/1 -> Bus Creator/9  "idxda"
  (delta)1/2 -> Bus Creator/10  "fda"

== system Test_Harness/Flight Dynamics/DATCOM Model/ToBus ==
  I : Inport
  Bus Creator3 : BusCreator  Inputs=3
  Demux : Demux  Outputs=3
  O : Outport
  wires:
  I/1 -> Demux/1
  Demux/2 -> Bus Creator3/2  "q_wind"
  Bus Creator3/1 -> O/1
  Demux/3 -> Bus Creator3/3  "r_wind"
  Demux/1 -> Bus Creator3/1  "p_wind"

== system Test_Harness/Secondary Arduino/Telemetry Logging/SD Logging ==

== system Test_Harness/Secondary Arduino/Telemetry Logging/Simulink Logging ==
  Telemetry : Inport
  Body Angles : Scope  NumInputPorts=3
  Body Velocities : Scope  NumInputPorts=3
  Bus Selector : BusSelector  OutputSignals=phi_theta_psi,V_b
  Demux : Demux  Outputs=3
  Demux1 : Demux  Outputs=3
  wires:
  Demux1/3 -> Body Velocities/3  "Z Vel"
  Demux1/2 -> Body Velocities/2  "Y Vel"
  Demux/3 -> Body Angles/3  "Yaw Angle"
  Demux/2 -> Body Angles/2  "Pitch Angle"
  Bus Selector/2 -> Demux1/1  "<V_b>"
  Bus Selector/1 -> Demux/1  "<phi_theta_psi>"
  Demux/1 -> Body Angles/1  "Roll Angle"
  Demux1/1 -> Body Velocities/1  "X Vel"
  Telemetry/1 -> Bus Selector/1

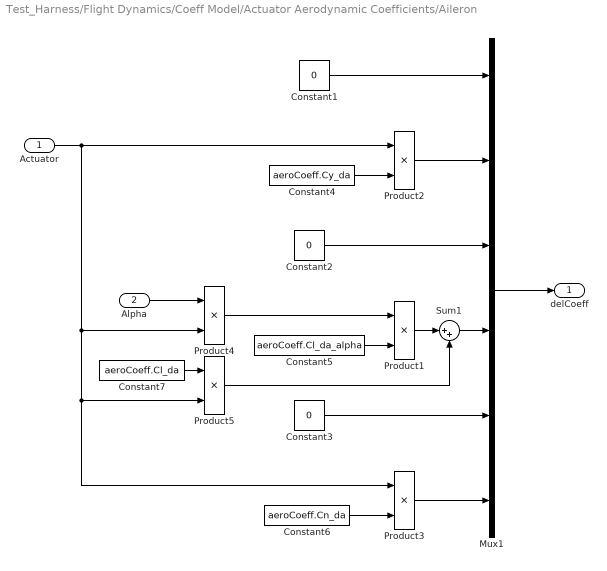
== system Test_Harness/Flight Dynamics/Coeff Model/Actuator Aerodynamic Coefficients/Aileron ==
  Actuator : Inport
  Alpha : Inport  Port=2
  Constant1 : Constant  Value=0
  Constant2 : Constant  Value=0
  Constant3 : Constant  Value=0
  Constant4 : Constant  Value=aeroCoeff.Cy_da
  Constant5 : Constant  Value=aeroCoeff.Cl_da_alpha
  Constant6 : Constant  Value=aeroCoeff.Cn_da
  Constant7 : Constant  Value=aeroCoeff.Cl_da
  Mux1 : Mux  Inputs=6
  Product{1..5} (5 alike) : Product  SaturateOnIntegerOverflow=on  InputSameDT=on  OutDataTypeStr=Inherit: Same as first input
  Sum1 : Sum  Inputs=|++
  delCoeff : Outport
  wires:
  Product5/1 -> Sum1/2
  Constant7/1 -> Product5/1
  Sum1/1 -> Mux1/4
  Product4/1 -> Product1/1
  Alpha/1 -> Product4/1
  Constant6/1 -> Product3/2
  Product3/1 -> Mux1/6
  Actuator/1 -> Product2/1, Product3/1, Product5/2, Product4/2
  Product1/1 -> Sum1/1
  Constant5/1 -> Product1/2
  Constant4/1 -> Product2/2
  Constant3/1 -> Mux1/5
  Constant2/1 -> Mux1/3
  Constant1/1 -> Mux1/1
  Mux1/1 -> delCoeff/1
  Product2/1 -> Mux1/2

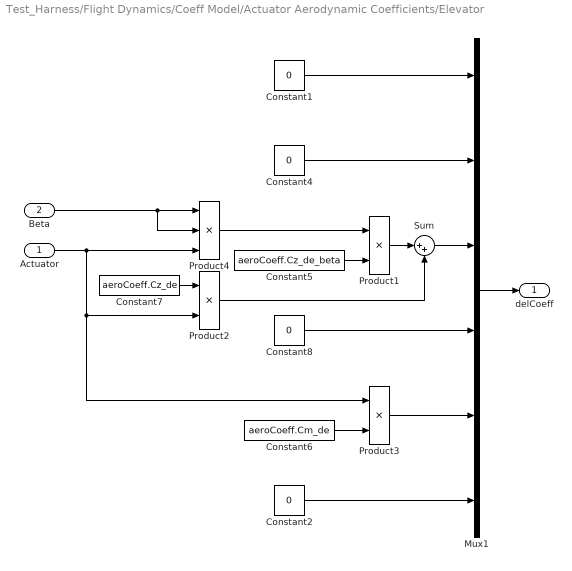
== system Test_Harness/Flight Dynamics/Coeff Model/Actuator Aerodynamic Coefficients/Elevator ==
  Actuator : Inport
  Beta : Inport  Port=2
  Constant{1..2,4,8} (4 alike) : Constant  Value=0
  Constant5 : Constant  Value=aeroCoeff.Cz_de_beta
  Constant6 : Constant  Value=aeroCoeff.Cm_de
  Constant7 : Constant  Value=aeroCoeff.Cz_de
  Mux1 : Mux  Inputs=6
  Product1 : Product  SaturateOnIntegerOverflow=on  InputSameDT=on  OutDataTypeStr=Inherit: Same as first input
  Product2 : Product  SaturateOnIntegerOverflow=on  InputSameDT=on  OutDataTypeStr=Inherit: Same as first input
  Product3 : Product  SaturateOnIntegerOverflow=on  InputSameDT=on  OutDataTypeStr=Inherit: Same as first input
  Product4 : Product  Inputs=3  SaturateOnIntegerOverflow=on  InputSameDT=on  OutDataTypeStr=Inherit: Same as first input
  Sum : Sum  Inputs=|++
  delCoeff : Outport
  wires:
  Product2/1 -> Sum/2
  Beta/1 -> Product4/1, Product4/2
  Product3/1 -> Mux1/5
  Constant2/1 -> Mux1/6
  Constant8/1 -> Mux1/4
  Constant1/1 -> Mux1/1
  Product1/1 -> Sum/1
  Mux1/1 -> delCoeff/1
  Constant4/1 -> Mux1/2
  Constant7/1 -> Product2/1
  Product4/1 -> Product1/1
  Constant5/1 -> Product1/2
  Constant6/1 -> Product3/2
  Actuator/1 -> Product4/3, Product2/2, Product3/1
  Sum/1 -> Mux1/3

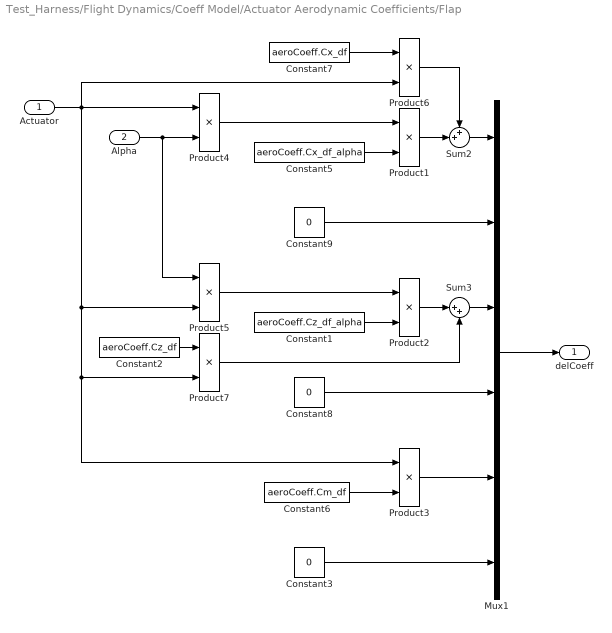
== system Test_Harness/Flight Dynamics/Coeff Model/Actuator Aerodynamic Coefficients/Flap ==
  Actuator : Inport
  Alpha : Inport  Port=2
  Constant1 : Constant  Value=aeroCoeff.Cz_df_alpha
  Constant2 : Constant  Value=aeroCoeff.Cz_df
  Constant3 : Constant  Value=0
  Constant5 : Constant  Value=aeroCoeff.Cx_df_alpha
  Constant6 : Constant  Value=aeroCoeff.Cm_df
  Constant7 : Constant  Value=aeroCoeff.Cx_df
  Constant8 : Constant  Value=0
  Constant9 : Constant  Value=0
  Mux1 : Mux  Inputs=6
  Product{1..7} (7 alike) : Product  SaturateOnIntegerOverflow=on  InputSameDT=on  OutDataTypeStr=Inherit: Same as first input
  Sum2 : Sum  Inputs=++|
  Sum3 : Sum  Inputs=|++
  delCoeff : Outport
  wires:
  Product7/1 -> Sum3/2
  Product6/1 -> Sum2/1
  Product1/1 -> Sum2/2
  Constant1/1 -> Product2/2
  Product5/1 -> Product2/1
  Alpha/1 -> Product5/1, Product4/2
  Constant2/1 -> Product7/1
  Product2/1 -> Sum3/1
  Sum3/1 -> Mux1/3
  Sum2/1 -> Mux1/1
  Product3/1 -> Mux1/5
  Constant9/1 -> Mux1/2
  Constant8/1 -> Mux1/4
  Mux1/1 -> delCoeff/1
  Constant3/1 -> Mux1/6
  Constant7/1 -> Product6/1
  Product4/1 -> Product1/1
  Constant5/1 -> Product1/2
  Constant6/1 -> Product3/2
  Actuator/1 -> Product4/1, Product7/2, Product3/1, Product5/2, Product6/2

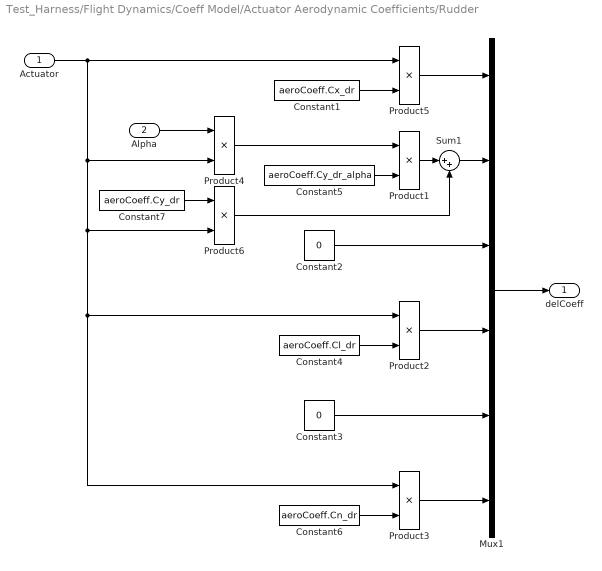
== system Test_Harness/Flight Dynamics/Coeff Model/Actuator Aerodynamic Coefficients/Rudder ==
  Actuator : Inport
  Alpha : Inport  Port=2
  Constant1 : Constant  Value=aeroCoeff.Cx_dr
  Constant2 : Constant  Value=0
  Constant3 : Constant  Value=0
  Constant4 : Constant  Value=aeroCoeff.Cl_dr
  Constant5 : Constant  Value=aeroCoeff.Cy_dr_alpha
  Constant6 : Constant  Value=aeroCoeff.Cn_dr
  Constant7 : Constant  Value=aeroCoeff.Cy_dr
  Mux1 : Mux  Inputs=6
  Product{1..6} (6 alike) : Product  SaturateOnIntegerOverflow=on  InputSameDT=on  OutDataTypeStr=Inherit: Same as first input
  Sum1 : Sum  Inputs=|++
  delCoeff : Outport
  wires:
  Product6/1 -> Sum1/2
  Sum1/1 -> Mux1/2
  Product5/1 -> Mux1/1
  Constant1/1 -> Product5/2
  Product2/1 -> Mux1/4
  Product3/1 -> Mux1/6
  Constant4/1 -> Product2/2
  Product1/1 -> Sum1/1
  Mux1/1 -> delCoeff/1
  Constant3/1 -> Mux1/5
  Constant7/1 -> Product6/1
  Constant2/1 -> Mux1/3
  Alpha/1 -> Product4/1
  Product4/1 -> Product1/1
  Constant5/1 -> Product1/2
  Constant6/1 -> Product3/2
  Actuator/1 -> Product5/1, Product4/2, Product6/2, Product2/1, Product3/1

== system Test_Harness/Flight Dynamics/Coeff Model/Aerodynamic Coefficients/Body Rate Damping ==
  V : Inport  Unit=m/s
  Bus Element In : Inport  Port=2  PortName=pqr  Element=p_wind
  Bus Element In1 : Inport  Port=2  PortName=pqr  Element=q_wind
  Bus Element In2 : Inport  Port=2  PortName=pqr  Element=r_wind
  Product : Product  SaturateOnIntegerOverflow=on  InputSameDT=on  OutDataTypeStr=Inherit: Same as first input
  Product1 : Product  SaturateOnIntegerOverflow=on  InputSameDT=on  OutDataTypeStr=Inherit: Same as first input
  Product2 : Product  SaturateOnIntegerOverflow=on  InputSameDT=on  OutDataTypeStr=Inherit: Same as first input
  Product3 : Product  Inputs=*/  SaturateOnIntegerOverflow=on  InputSameDT=on  OutDataTypeStr=Inherit: Same as first input
  Reference Length : Gain  Gain=vehicle.chord  SaturateOnIntegerOverflow=on  OutDataTypeStr=Inherit: Same as input  ParamDataTypeStr=Inherit: Same as input
  Reference Span : Gain  Gain=vehicle.wingspan/2  SaturateOnIntegerOverflow=on  OutDataTypeStr=Inherit: Same as input  ParamDataTypeStr=Inherit: Same as input
  "Reference Span " : Gain  Gain=vehicle.wingspan/2  SaturateOnIntegerOverflow=on  OutDataTypeStr=Inherit: Same as input  ParamDataTypeStr=Inherit: Same as input
  Sum1 : Sum  Inputs=+++  SaturateOnIntegerOverflow=on  InputSameDT=on  OutDataTypeStr=Inherit: Same as first input
  p : Subsystem
  q : Subsystem
  r : Subsystem
  Coeff : Outport  InitialOutput=0
  wires:
  Bus Element In/1 -> Product/2
  Bus Element In1/1 -> Product1/2
  Bus Element In2/1 -> Product2/2
  p/1(delCoeff) -> Product/1
  q/1(delCoeff) -> Product1/1
  Sum1/1 -> Product3/1
  V/1 -> Product3/2
  Product3/1 -> Coeff/1
  Product1/1 -> Reference Length/1
  Product2/1 -> "Reference Span "/1
  Product/1 -> Reference Span/1
  r/1(delCoeff) -> Product2/1
  Reference Length/1 -> Sum1/2
  Reference Span/1 -> Sum1/1
  "Reference Span "/1 -> Sum1/3

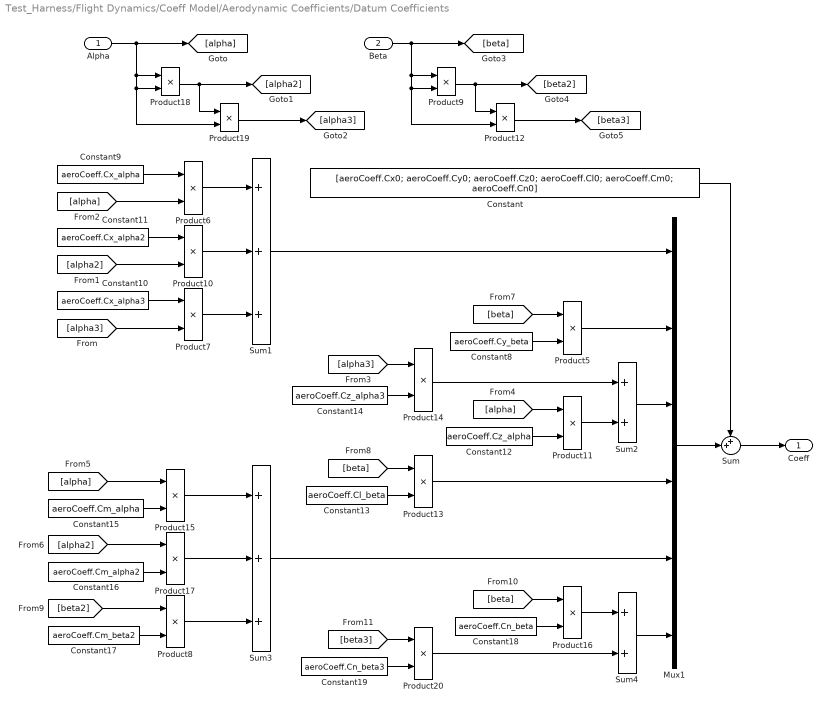
== system Test_Harness/Flight Dynamics/Coeff Model/Aerodynamic Coefficients/Datum Coefficients ==
  Alpha : Inport
  Beta : Inport  Port=2
  Constant : Constant  Value=[aeroCoeff.Cx0; aeroCoeff.Cy0; aeroCoeff.Cz0; aeroCoeff.Cl0; aeroCoeff.Cm0; aeroCoeff.Cn0]
  Constant10 : Constant  Value=aeroCoeff.Cx_alpha3
  Constant11 : Constant  Value=aeroCoeff.Cx_alpha2
  Constant12 : Constant  Value=aeroCoeff.Cz_alpha
  Constant13 : Constant  Value=aeroCoeff.Cl_beta
  Constant14 : Constant  Value=aeroCoeff.Cz_alpha3
  Constant15 : Constant  Value=aeroCoeff.Cm_alpha
  Constant16 : Constant  Value=aeroCoeff.Cm_alpha2
  Constant17 : Constant  Value=aeroCoeff.Cm_beta2
  Constant18 : Constant  Value=aeroCoeff.Cn_beta
  Constant19 : Constant  Value=aeroCoeff.Cn_beta3
  Constant8 : Constant  Value=aeroCoeff.Cy_beta
  Constant9 : Constant  Value=aeroCoeff.Cx_alpha
  Mux1 : Mux  Inputs=6
  Product{5..20} (16 alike) : Product  SaturateOnIntegerOverflow=on  InputSameDT=on  OutDataTypeStr=Inherit: Same as first input
  Sum : Sum  Inputs=++|
  Sum1 : Sum  Inputs=+++  SaturateOnIntegerOverflow=on
  Sum2 : Sum  Inputs=2  SaturateOnIntegerOverflow=on
  Sum3 : Sum  Inputs=+++  SaturateOnIntegerOverflow=on
  Sum4 : Sum  Inputs=2  SaturateOnIntegerOverflow=on
  Coeff : Outport  InitialOutput=0
  wires:
  Sum/1 -> Coeff/1
  Constant/1 -> Sum/1
  Mux1/1 -> Sum/2
  Sum3/1 -> Mux1/5
  Product16/1 -> Sum4/1
  Product20/1 -> Sum4/2
  [beta3] -> Product20/1
  [beta] -> Product16/1
  Constant19/1 -> Product20/2
  Constant18/1 -> Product16/2
  Sum4/1 -> Mux1/6
  [beta2] -> Product8/1
  [beta] -> Product13/1
  [beta] -> Product5/1
  Beta/1 -> Product9/1, Product12/2, Product9/2, [beta]
  Product9/1 -> Product12/1, [beta2]
  Product12/1 -> [beta3]
  Product8/1 -> Sum3/3
  Constant17/1 -> Product8/2
  [alpha] -> Product15/1
  [alpha] -> Product11/1
  [alpha3] -> Product14/1
  [alpha] -> Product6/2
  [alpha2] -> Product10/2
  Constant10/1 -> Product7/1
  [alpha3] -> Product7/2
  Product19/1 -> [alpha3]
  Product18/1 -> [alpha2], Product19/1
  Alpha/1 -> [alpha], Product18/2, Product19/2, Product18/1
  Constant16/1 -> Product17/2
  Product17/1 -> Sum3/2
  [alpha2] -> Product17/1
  Constant15/1 -> Product15/2
  Product15/1 -> Sum3/1
  Constant14/1 -> Product14/2
  Product13/1 -> Mux1/4
  Constant13/1 -> Product13/2
  Sum2/1 -> Mux1/3
  Product14/1 -> Sum2/1
  Product11/1 -> Sum2/2
  Constant12/1 -> Product11/2
  Product10/1 -> Sum1/2
  Product6/1 -> Sum1/1
  Product7/1 -> Sum1/3
  Constant11/1 -> Product10/1
  Constant9/1 -> Product6/1
  Sum1/1 -> Mux1/1
  Product5/1 -> Mux1/2
  Constant8/1 -> Product5/2

== system Test_Harness/Flight Dynamics/DATCOM Model/Aero Coeffs/Aileron ==
  Bus : Inport
  Bus Selector2 : BusSelector  OutputSignals=idxa,fa,idxda,fda,idxm,fm,idxh,fh
  Bus Selector3 : BusSelector  OutputSignals=idxda,fda,idxm,fm,idxh,fh
  Constant1 : Constant  Value=0
  DCL_Roll : Interpolation_n-D  NumberOfTableDimensions=3  Table="permute(datcom1{2}.clroll,[1  2  3])"  RemoveProtectionIndex=on
      settings: InputPortMap=u0,u1,u2,u3,u4,u5
  DCN_Asym : Interpolation_n-D  NumberOfTableDimensions=4  Table=permute(datcom1{2}.cn_asy,[1 2 3 4 ])  RemoveProtectionIndex=on
      settings: InputPortMap=u0,u1,u2,u3,u4,u5,u6,u7
  Mux1 : Mux  Inputs=6
  delCoeff : Outport
  wires:
  Mux1/1 -> delCoeff/1
  Bus Selector3/5 -> DCL_Roll/5  "<idxh>"
  Constant1/1 -> Mux1/1, Mux1/2, Mux1/3, Mux1/5
  Bus Selector3/4 -> DCL_Roll/4  "<fm>"
  Bus Selector3/3 -> DCL_Roll/3  "<idxm>"
  Bus Selector3/6 -> DCL_Roll/6  "<fh>"
  Bus Selector3/1 -> DCL_Roll/1  "<idxda>"
  Bus Selector3/2 -> DCL_Roll/2  "<fda>"
  Bus Selector2/2 -> DCN_Asym/2  "<fa>"
  Bus Selector2/1 -> DCN_Asym/1  "<idxa>"
  Bus/1 -> Bus Selector2/1, Bus Selector3/1
  Bus Selector2/3 -> DCN_Asym/3  "<idxda>"
  Bus Selector2/4 -> DCN_Asym/4  "<fda>"
  Bus Selector2/5 -> DCN_Asym/5  "<idxm>"
  Bus Selector2/6 -> DCN_Asym/6  "<fm>"
  Bus Selector2/7 -> DCN_Asym/7  "<idxh>"
  Bus Selector2/8 -> DCN_Asym/8  "<fh>"
  DCN_Asym/1 -> Mux1/6
  DCL_Roll/1 -> Mux1/4

== system Test_Harness/Flight Dynamics/DATCOM Model/Aero Coeffs/Elevator ==
  Bus : Inport
  Bus Selector2 : BusSelector  OutputSignals=idxa,fa,idxm,fm,idxh,fh,idxde,fde
  Bus Selector3 : BusSelector  OutputSignals=idxde,fde,idxm,fm,idxh,fh
  Bus Selector5 : BusSelector  OutputSignals=idxde,fde,idxm,fm,idxh,fh
  Constant1 : Constant  Value=0
  DCDI : Interpolation_n-D  NumberOfTableDimensions=4  Table=permute(datcom1{3}.dcdi_sym,[1 3 4 2 ])  RemoveProtectionIndex=on
      settings: InputPortMap=u0,u1,u2,u3,u4,u5,u6,u7
  DCL : Interpolation_n-D  NumberOfTableDimensions=3  Table="permute(datcom1{3}.dcl_sym,[1  2  3])"  RemoveProtectionIndex=on
      settings: InputPortMap=u0,u1,u2,u3,u4,u5
  DCm : Interpolation_n-D  NumberOfTableDimensions=3  Table="permute(datcom1{3}.dcm_sym,[1  2  3])"  RemoveProtectionIndex=on
      settings: InputPortMap=u0,u1,u2,u3,u4,u5
  Mux1 : Mux  Inputs=6
  delCoeff : Outport
  wires:
  Mux1/1 -> delCoeff/1
  Bus/1 -> Bus Selector2/1, Bus Selector3/1, Bus Selector5/1
  DCDI/1 -> Mux1/1
  DCL/1 -> Mux1/3
  DCm/1 -> Mux1/5
  Constant1/1 -> Mux1/2, Mux1/4, Mux1/6
  Bus Selector2/1 -> DCDI/1  "<idxa>"
  Bus Selector2/2 -> DCDI/2  "<fa>"
  Bus Selector3/1 -> DCL/1  "<idxde>"
  Bus Selector3/2 -> DCL/2  "<fde>"
  Bus Selector5/1 -> DCm/1  "<idxde>"
  Bus Selector5/2 -> DCm/2  "<fde>"
  Bus Selector2/3 -> DCDI/3  "<idxm>"
  Bus Selector2/4 -> DCDI/4  "<fm>"
  Bus Selector2/5 -> DCDI/5  "<idxh>"
  Bus Selector2/6 -> DCDI/6  "<fh>"
  Bus Selector2/7 -> DCDI/7  "<idxde>"
  Bus Selector2/8 -> DCDI/8  "<fde>"
  Bus Selector3/3 -> DCL/3  "<idxm>"
  Bus Selector3/4 -> DCL/4  "<fm>"
  Bus Selector3/5 -> DCL/5  "<idxh>"
  Bus Selector3/6 -> DCL/6  "<fh>"
  Bus Selector5/3 -> DCm/3  "<idxm>"
  Bus Selector5/4 -> DCm/4  "<fm>"
  Bus Selector5/5 -> DCm/5  "<idxh>"
  Bus Selector5/6 -> DCm/6  "<fh>"

== system Test_Harness/Flight Dynamics/DATCOM Model/Aero Coeffs/Rudder ==
  Bus : Inport
  Constant1 : Constant  Value=0
  Mux1 : Mux  Inputs=6
  Terminator : Terminator
  delCoeff : Outport
  wires:
  Mux1/1 -> delCoeff/1
  Constant1/1 -> Mux1/6, Mux1/5, Mux1/4, Mux1/3, Mux1/2, Mux1/1
  Bus/1 -> Terminator/1

== system Test_Harness/Flight Dynamics/Coeff Model/Aerodynamic Coefficients/Body Rate Damping/p ==
  Constant1 : Constant  Value=0
  Constant2 : Constant  Value=0
  Constant3 : Constant  Value=0
  Constant4 : Constant  Value=aeroCoeff.Cl_p
  Constant5 : Constant  Value=aeroCoeff.Cn_p
  Constant8 : Constant  Value=aeroCoeff.Cy_p
  Mux1 : Mux  Inputs=6
  delCoeff : Outport
  wires:
  Constant4/1 -> Mux1/4
  Constant5/1 -> Mux1/6
  Constant8/1 -> Mux1/2
  Constant2/1 -> Mux1/3
  Constant3/1 -> Mux1/5
  Constant1/1 -> Mux1/1
  Mux1/1 -> delCoeff/1

== system Test_Harness/Flight Dynamics/Coeff Model/Aerodynamic Coefficients/Body Rate Damping/q ==
  Constant1 : Constant  Value=0
  Constant2 : Constant  Value=0
  Constant3 : Constant  Value=aeroCoeff.Cn_q
  Constant4 : Constant  Value=aeroCoeff.Cz_q
  Constant5 : Constant  Value=aeroCoeff.Cm_q
  Constant8 : Constant  Value=aeroCoeff.Cx_q
  Mux1 : Mux  Inputs=6
  delCoeff : Outport
  wires:
  Constant3/1 -> Mux1/6
  Constant5/1 -> Mux1/5
  Constant4/1 -> Mux1/3
  Constant8/1 -> Mux1/1
  Constant1/1 -> Mux1/2
  Constant2/1 -> Mux1/4
  Mux1/1 -> delCoeff/1

== system Test_Harness/Flight Dynamics/Coeff Model/Aerodynamic Coefficients/Body Rate Damping/r ==
  Constant1 : Constant  Value=0
  Constant2 : Constant  Value=0
  Constant3 : Constant  Value=aeroCoeff.Cm_r
  Constant4 : Constant  Value=aeroCoeff.Cl_r
  Constant5 : Constant  Value=aeroCoeff.Cn_r
  Constant6 : Constant  Value=aeroCoeff.Cy_r
  Mux1 : Mux  Inputs=6
  delCoeff : Outport
  wires:
  Constant6/1 -> Mux1/2
  Constant2/1 -> Mux1/3
  Constant3/1 -> Mux1/5
  Constant5/1 -> Mux1/6
  Constant1/1 -> Mux1/1
  Mux1/1 -> delCoeff/1
  Constant4/1 -> Mux1/4
